simulink model "sys_noisy"  (R2018b)
settings: Solver=VariableStepAuto  StartTime=0.0  StopTime=10  RelTol=1e-6
undefined symbols (not defined in the file): A, B, B1, C, D, K, L
libraries: simulink x2
settings Model: Creator=1  LastModifiedBy=1

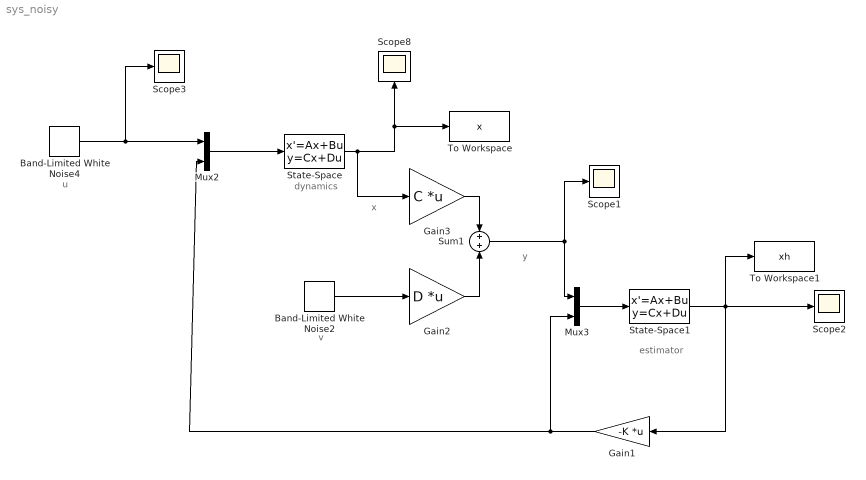
== system sys_noisy ==
  note: x
  note: y
  note: estimator
  note: dynamics
  note: v
  note: u
  Band-Limited White Noise2 : simulink/Sources/Band-Limited White Noise  Cov=[0.1]  Ts=0.1  seed=[23343; 23344]  VectorParams1D=off
  Band-Limited White Noise4 : simulink/Sources/Band-Limited White Noise  Cov=[0.1]  Ts=0.1  seed=[23341;23342]  VectorParams1D=off
  Gain1 : Gain  Gain=-K  Multiplication=Matrix(K*u)
  Gain2 : Gain  Gain=D  Multiplication=Matrix(K*u)
  Gain3 : Gain  Gain=C  Multiplication=Matrix(K*u)
  Mux2 : Mux  Inputs=2
  Mux3 : Mux  Inputs=2
  Scope{1..3,8} (4 alike) : Scope
  State-Space : StateSpace  A=A  B=[B B1]  C=eye(4)  D=zeros(4,3)  InitialCondition=[0,0,0,0]
  State-Space1 : StateSpace  A=A-L*C  B=[L B1]  C=eye(4)  D=zeros(4,3)  InitialCondition=[0,0,0,0]
  Sum1 : Sum  Inputs=+|+
  To Workspace : ToWorkspace  VariableName=x  SaveFormat=Timeseries  SampleTime=-1
  To Workspace1 : ToWorkspace  VariableName=xh  SaveFormat=Timeseries  SampleTime=-1
  wires:
  State-Space/1 -> To Workspace/1, Scope8/1, Gain3/1
  Gain2/1 -> Sum1/2
  Band-Limited White Noise2/1 -> Gain2/1
  Gain3/1 -> Sum1/1
  Sum1/1 -> Scope1/1, Mux3/1
  Mux3/1 -> State-Space1/1
  State-Space1/1 -> To Workspace1/1, Gain1/1, Scope2/1
  Band-Limited White Noise4/1 -> Scope3/1, Mux2/1
  Mux2/1 -> State-Space/1
  Gain1/1 -> Mux3/2, Mux2/2
